simulink model "Progetto_robotics_linear"  (R2021a)
settings: Solver=ode4  StartTime=0.0  StopTime=Tsim_lin  FixedStep=Ts  RelTol=1e-3
InitFcn:
  | I1=1;
  | I2=2;
  | I3 =3;
values from neighbouring files (symbols this model uses):
  q_iniz_lin = [-pi/4;+3/4*pi;-3/4*pi]    [File_main_lineare.m]
(part 1 of 2)
settings Model: Creator=lorenzomaiani  LastModifiedBy=lorenzomaiani

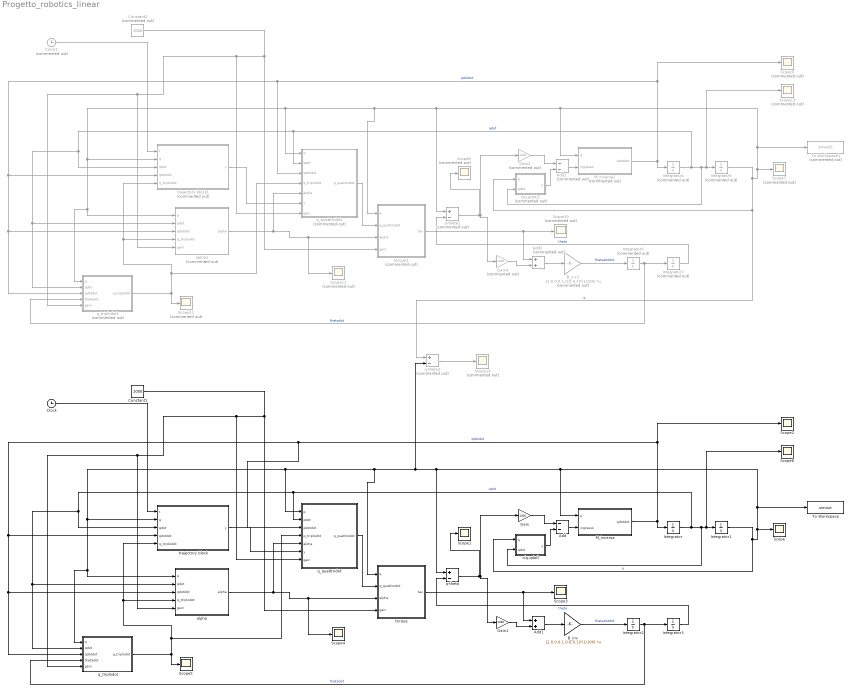
== system Progetto_robotics_linear ==
  "  M_inversa" : MATLAB Function  TreatAsAtomicUnit=on
  "  M_inversa1" : MATLAB Function  Commented=on  TreatAsAtomicUnit=on
  " c(q,qdot)" : MATLAB Function  TreatAsAtomicUnit=on
  " c(q,qdot)1" : MATLAB Function  Commented=on  TreatAsAtomicUnit=on
  Add : Sum  Inputs=--
  Add1 : Sum
  Add2 : Sum  Commented=on  Inputs=--
  Add3 : Sum  Commented=on
  B_inv : Gain  Gain=[1,0,0;0,1,0;0,0,1]*(1/100)  Multiplication=Matrix(K*u) (u vector)
  B_inv1 : Gain  Commented=on  Gain=[1,0,0;0,1,0;0,0,1]*(1/100)  Multiplication=Matrix(K*u) (u vector)
  Clock : Clock
  Clock1 : Clock  Commented=on
  Constant1 : Constant  Value=1000
  Constant2 : Constant  Commented=on  Value=1000
  Gain : Gain  Gain=1000
  Gain1 : Gain  Gain=1000
  Gain2 : Gain  Commented=on  Gain=1000
  Gain3 : Gain  Commented=on  Gain=1000
  Integrator : Integrator  InitialCondition=[0;0;0]
  Integrator1 : Integrator  InitialCondition=q_iniz_lin
  Integrator2 : Integrator  InitialCondition=[0;0;0]
  Integrator3 : Integrator  InitialCondition=q_iniz_lin
  Integrator4 : Integrator  Commented=on  InitialCondition=[0;0;0]
  Integrator5 : Integrator  Commented=on  InitialCondition=q_iniz_lin
  Integrator6 : Integrator  Commented=on  InitialCondition=[0;0;0]
  Integrator7 : Integrator  Commented=on  InitialCondition=q_iniz_lin
  Scope{,1..6} (7 alike) : Scope
  Scope{7..14} (8 alike) : Scope  Commented=on
  To Workspace : ToWorkspace  VariableName=simout  SampleTime=-1
  To Workspace1 : ToWorkspace  Commented=on  VariableName=simout1  SampleTime=-1
  alpha : MATLAB Function  TreatAsAtomicUnit=on
  alpha1 : MATLAB Function  Commented=on  TreatAsAtomicUnit=on
  q-theta : Sum  Inputs=+-
  q-theta1 : Sum  Commented=on  Inputs=+-
  q-theta2 : Sum  Commented=on  Inputs=+-
  q_quattrodot : MATLAB Function  TreatAsAtomicUnit=on
  q_quattrodot1 : MATLAB Function  Commented=on  TreatAsAtomicUnit=on
  q_triplodot : MATLAB Function  TreatAsAtomicUnit=on
  q_triplodot1 : MATLAB Function  Commented=on  TreatAsAtomicUnit=on
  torque : MATLAB Function  TreatAsAtomicUnit=on
  torque1 : MATLAB Function  Commented=on  TreatAsAtomicUnit=on
  trajectory block : MATLAB Function  TreatAsAtomicUnit=on
  trajectory block1 : MATLAB Function  Commented=on  TreatAsAtomicUnit=on
  wires:
  Integrator/1 -> q_quattrodot/2(qdot), q_triplodot/2(qdot), alpha/2(qdot), trajectory block/3(qdot), " c(q,qdot)"/2(qdot), Scope6/1, Integrator1/1  "qdot"
  Integrator1/1 -> To Workspace/1, "  M_inversa"/1(q), q-theta2/2, torque/1(q), q_quattrodot/1(q), alpha/1(q), q_triplodot/1(q), trajectory block/2(q), q-theta/1, Scope/1, " c(q,qdot)"/1(q)  "q"
  "  M_inversa"/1(qdotdot) -> Scope2/1, q_quattrodot/3(qdotdot), q_triplodot/3(qdotdot), alpha/3(qdotdot), trajectory block/4(qdotdot), Integrator/1  "qdotdot"
  " c(q,qdot)"/1(y) -> Add/2
  Gain/1 -> Add/1
  Integrator3/1 -> q-theta/2  "theta"
  Integrator2/1 -> q_triplodot/4(thetadot), Integrator3/1  "thetadot"
  Add1/1 -> B_inv/1
  Gain1/1 -> Add1/2
  q_quattrodot/1(q_quattrodot) -> torque/2(q_quattrodot)
  alpha/1(alpha) -> Scope4/1, torque/3(alpha), q_quattrodot/5(alpha)
  q_triplodot/1(q_triplodot) -> q_quattrodot/4(q_triplodot), trajectory block/5(q_triplodot), alpha/4(q_triplodot), Scope5/1
  trajectory block/1(y) -> q_quattrodot/6(y)
  Clock/1 -> trajectory block/1(t)
  Add/1 -> "  M_inversa"/2(ingresso)
  B_inv/1 -> Integrator2/1  "thetadotdot"
  Constant1/1 -> alpha/5(gain), q_triplodot/5(gain), q_quattrodot/7(gain), torque/4(gain)
  q-theta/1 -> Scope1/1, Gain/1, Gain1/1
  torque/1(tau) -> Scope3/1, Add1/1
  Gain2/1 -> Add2/1
  "  M_inversa1"/1(qdotdot) -> Scope9/1, q_quattrodot1/3(qdotdot), q_triplodot1/3(qdotdot), alpha1/3(qdotdot), trajectory block1/4(qdotdot), Integrator4/1  "qdotdot"
  alpha1/1(alpha) -> Scope11/1, torque1/3(alpha), q_quattrodot1/5(alpha)
  q-theta1/1 -> Scope8/1, Gain2/1, Gain3/1
  " c(q,qdot)1"/1(y) -> Add2/2
  Integrator7/1 -> q-theta1/2  "theta"
  Add3/1 -> B_inv1/1
  Constant2/1 -> alpha1/5(gain), q_triplodot1/5(gain), q_quattrodot1/7(gain), torque1/4(gain)
  Integrator5/1 -> To Workspace1/1, "  M_inversa1"/1(q), torque1/1(q), q_quattrodot1/1(q), alpha1/1(q), q_triplodot1/1(q), trajectory block1/2(q), q-theta1/1, Scope7/1, q-theta2/1, " c(q,qdot)1"/1(q)  "q"
  trajectory block1/1(y) -> q_quattrodot1/6(y)
  torque1/1(tau) -> Scope10/1, Add3/1
  Integrator6/1 -> q_triplodot1/4(thetadot), Integrator7/1  "thetadot"
  B_inv1/1 -> Integrator6/1  "thetadotdot"
  Integrator4/1 -> q_quattrodot1/2(qdot), q_triplodot1/2(qdot), alpha1/2(qdot), trajectory block1/3(qdot), " c(q,qdot)1"/2(qdot), Scope13/1, Integrator5/1  "qdot"
  q_triplodot1/1(q_triplodot) -> q_quattrodot1/4(q_triplodot), trajectory block1/5(q_triplodot), alpha1/4(q_triplodot), Scope12/1
  Gain3/1 -> Add3/2
  Clock1/1 -> trajectory block1/1(t)
  Add2/1 -> "  M_inversa1"/2(ingresso)
  q_quattrodot1/1(q_quattrodot) -> torque1/2(q_quattrodot)
  q-theta2/1 -> Scope14/1

== matlab function Progetto_robotics_linear/ c(q,qdot)1 ==
  data: q input; y output; qdot input
function y = fcn(q,qdot)


q1=q(1);
q2=q(2);
q3=q(3);

q1_dot=qdot(1);
q2_dot=qdot(2);
q3_dot=qdot(3);




c=[- q1_dot*(q3_dot*(5*sin(q2 + q3) + 5*sin(q3)) + q2_dot*(5*sin(q2 + q3) + 16*sin(q2))) - q3_dot*(q1_dot*(5*sin(q2 + q3) + 5*sin(q3)) + q2_dot*(5*sin(q2 + q3) + 5*sin(q3)) + q3_dot*(5*sin(q2 + q3) + 5*sin(q3))) - q2_dot*(q3_dot*(5*sin(q2 + q3) + 5*sin(q3)) + q2_dot*(5*sin(q2 + q3) + 11*sin(q2)) + q1_dot*(5*sin(q2 + q3) + 16*sin(q2)));
                                                                                                                                                                                q1_dot*(q1_dot*(5*sin(q2 + q3) + 16*sin(q2)) - 5*q3_dot*sin(q3)) - q3_dot*(5*q1_dot*sin(q3) + 5*q2_dot*sin(q3) + 10*q3_dot*sin(q3)) - 5*q2_dot*q3_dot*sin(q3);
                                                                                                                                                                                                                               q1_dot*(q1_dot*(5*sin(q2 + q3) + 5*sin(q3)) + 5*q2_dot*sin(q3)) + q2_dot*(5*q1_dot*sin(q3) + 5*q2_dot*sin(q3))];
                                                                                                                                                                                                                                                                                                                                                         
                                                                                                                                                                                                                                                                                                                                                            
                                                                                                                                                                                                                                                                                                                                                            
y = c;

== matlab function Progetto_robotics_linear/alpha1 ==
  data: q input; alpha output; qdot input; qdotdot input; q_triplodot input; gain input
function alpha = fcn(q,qdot,qdotdot,q_triplodot,gain)

q1=q(1);
q2=q(2);
q3=q(3);

q1_dot=qdot(1);
q2_dot=qdot(2);
q3_dot=qdot(3);

q1_dotdot=qdotdot(1);
q2_dotdot=qdotdot(2);
q3_dotdot=qdotdot(3);

%usare per blocco jacobiano
q1_tridot=q_triplodot(1);
q2_tridot=q_triplodot(2);
q3_tridot=q_triplodot(3);


K=gain*eye(3);
B=100*[1,0,0;0,1,0;0,0,1];


%M matrix
m=[10*cos(q2 + q3) + 32*cos(q2) + 10*cos(q3) + 5049/100, 5*cos(q2 + q3) + 11*cos(q2) + 10*cos(q3) + 504/25, 5*cos(q2 + q3) + 5*cos(q3) + 583/100;
   5*cos(q2 + q3) + 11*cos(q2) + 10*cos(q3) + 504/25,                              10*cos(q3) + 1133/50,                 10*cos(q3) + 583/100;
                5*cos(q2 + q3) + 5*cos(q3) + 583/100,                              10*cos(q3) + 583/100,                              583/100];



%coriolis and centrif.
c=[- q1_dot*(q3_dot*(5*sin(q2 + q3) + 5*sin(q3)) + q2_dot*(5*sin(q2 + q3) + 16*sin(q2))) - q3_dot*(q1_dot*(5*sin(q2 + q3) + 5*sin(q3)) + q2_dot*(5*sin(q2 + q3) + 5*sin(q3)) + q3_dot*(5*sin(q2 + q3) + 5*sin(q3))) - q2_dot*(q3_dot*(5*sin(q2 + q3) + 5*sin(q3)) + q2_dot*(5*sin(q2 + q3) + 11*sin(q2)) + q1_dot*(5*sin(q2 + q3) + 16*sin(q2)));
                                                                                                                                                                                q1_dot*(q1_dot*(5*sin(q2 + q3) + 16*sin(q2)) - 5*q3_dot*sin(q3)) - q3_dot*(5*q1_dot*sin(q3) + 5*q2_dot*sin(q3) + 10*q3_dot*sin(q3)) - 5*q2_dot*q3_dot*sin(q3);
                                                                                                                                                                                                                               q1_dot*(q1_dot*(5*sin(q2 + q3) + 5*sin(q3)) + 5*q2_dot*sin(q3)) + q2_dot*(5*q1_dot*sin(q3) + 5*q2_dot*sin(q3))];



%coriolis and centrif. dotdot
cdotdot=[11*q2_dot^4*sin(q2) + 5*q3_dot^4*sin(q3) - 22*q2_dotdot^2*sin(q2) - 10*q3_dotdot^2*sin(q3) + 5*q2_dot^4*sin(q2 + q3) + 5*q3_dot^4*sin(q2 + q3) - 10*q2_dotdot^2*sin(q2 + q3) - 10*q3_dotdot^2*sin(q2 + q3) - 32*q1_dot*q2_tridot*sin(q2) - 32*q2_dot*q1_tridot*sin(q2) - 22*q2_dot*q2_tridot*sin(q2) - 10*q1_dot*q3_tridot*sin(q3) - 10*q3_dot*q1_tridot*sin(q3) - 10*q2_dot*q3_tridot*sin(q3) - 10*q3_dot*q2_tridot*sin(q3) - 10*q3_dot*q3_tridot*sin(q3) - 64*q1_dotdot*q2_dotdot*sin(q2) - 20*q1_dotdot*q3_dotdot*sin(q3) - 20*q2_dotdot*q3_dotdot*sin(q3) - 20*q2_dot^2*q1_dotdot*cos(q2 + q3) - 25*q2_dot^2*q2_dotdot*cos(q2 + q3) - 20*q3_dot^2*q1_dotdot*cos(q2 + q3) - 25*q2_dot^2*q3_dotdot*cos(q2 + q3) - 25*q3_dot^2*q2_dotdot*cos(q2 + q3) - 25*q3_dot^2*q3_dotdot*cos(q2 + q3) + 10*q1_dot*q2_dot^3*sin(q2 + q3) + 10*q1_dot*q3_dot^3*sin(q2 + q3) + 20*q2_dot*q3_dot^3*sin(q2 + q3) + 20*q2_dot^3*q3_dot*sin(q2 + q3) - 64*q2_dot^2*q1_dotdot*cos(q2) - 55*q2_dot^2*q2_dotdot*cos(q2) - 20*q3_dot^2*q1_dotdot*cos(q3) - 20*q3_dot^2*q2_dotdot*cos(q3) - 25*q3_dot^2*q3_dotdot*cos(q3) + 32*q1_dot*q2_dot^3*sin(q2) + 10*q1_dot*q3_dot^3*sin(q3) + 10*q2_dot*q3_dot^3*sin(q3) + 30*q2_dot^2*q3_dot^2*sin(q2 + q3) - 10*q1_dot*q2_tridot*sin(q2 + q3) - 10*q2_dot*q1_tridot*sin(q2 + q3) - 10*q1_dot*q3_tridot*sin(q2 + q3) - 10*q2_dot*q2_tridot*sin(q2 + q3) - 10*q3_dot*q1_tridot*sin(q2 + q3) - 10*q2_dot*q3_tridot*sin(q2 + q3) - 10*q3_dot*q2_tridot*sin(q2 + q3) - 10*q3_dot*q3_tridot*sin(q2 + q3) - 20*q1_dotdot*q2_dotdot*sin(q2 + q3) - 20*q1_dotdot*q3_dotdot*sin(q2 + q3) - 20*q2_dotdot*q3_dotdot*sin(q2 + q3) - 30*q1_dot*q2_dot*q2_dotdot*cos(q2 + q3) - 30*q1_dot*q2_dot*q3_dotdot*cos(q2 + q3) - 30*q1_dot*q3_dot*q2_dotdot*cos(q2 + q3) - 40*q2_dot*q3_dot*q1_dotdot*cos(q2 + q3) - 30*q1_dot*q3_dot*q3_dotdot*cos(q2 + q3) - 50*q2_dot*q3_dot*q2_dotdot*cos(q2 + q3) - 50*q2_dot*q3_dot*q3_dotdot*cos(q2 + q3) - 96*q1_dot*q2_dot*q2_dotdot*cos(q2) - 30*q1_dot*q3_dot*q3_dotdot*cos(q3) - 30*q2_dot*q3_dot*q3_dotdot*cos(q3) + 30*q1_dot*q2_dot*q3_dot^2*sin(q2 + q3) + 30*q1_dot*q2_dot^2*q3_dot*sin(q2 + q3);
                                                                                                                                                                                                                                                                                                                                                                                                                                                                                                                                                                                                                                                                                                                                                                                                                                                                                                                                                                                                                                                                                                                                10*q3_dot^4*sin(q3) + 32*q1_dotdot^2*sin(q2) - 20*q3_dotdot^2*sin(q3) + 10*q1_dotdot^2*sin(q2 + q3) + 32*q1_dot*q1_tridot*sin(q2) - 10*q1_dot*q3_tridot*sin(q3) - 10*q3_dot*q1_tridot*sin(q3) - 10*q2_dot*q3_tridot*sin(q3) - 10*q3_dot*q2_tridot*sin(q3) - 20*q3_dot*q3_tridot*sin(q3) - 20*q1_dotdot*q3_dotdot*sin(q3) - 20*q2_dotdot*q3_dotdot*sin(q3) + 5*q1_dot^2*q2_dotdot*cos(q2 + q3) + 5*q1_dot^2*q3_dotdot*cos(q2 + q3) + 16*q1_dot^2*q2_dotdot*cos(q2) - 20*q3_dot^2*q1_dotdot*cos(q3) - 20*q3_dot^2*q2_dotdot*cos(q3) - 50*q3_dot^2*q3_dotdot*cos(q3) + 10*q1_dot*q3_dot^3*sin(q3) + 10*q2_dot*q3_dot^3*sin(q3) - 5*q1_dot^2*q2_dot^2*sin(q2 + q3) - 5*q1_dot^2*q3_dot^2*sin(q2 + q3) - 16*q1_dot^2*q2_dot^2*sin(q2) + 10*q1_dot*q1_tridot*sin(q2 + q3) + 20*q1_dot*q2_dot*q1_dotdot*cos(q2 + q3) + 20*q1_dot*q3_dot*q1_dotdot*cos(q2 + q3) + 64*q1_dot*q2_dot*q1_dotdot*cos(q2) - 30*q1_dot*q3_dot*q3_dotdot*cos(q3) - 30*q2_dot*q3_dot*q3_dotdot*cos(q3) - 10*q1_dot^2*q2_dot*q3_dot*sin(q2 + q3);
                                                                                                                                                                                                                                                                                                                                                                                                                                                                                                                                                                                                                                                                                                                                                                                                                                                                                                                                                                                                                                                                                                                                                                                                                                                                                                                                                                                        10*q2_dotdot^2*sin(q3) + q1_tridot*(10*q1_dot*sin(q2 + q3) + 10*q1_dot*sin(q3) + 10*q2_dot*sin(q3)) + q3_dotdot*(5*q1_dot^2*cos(q3) + 5*q2_dot^2*cos(q3) + 5*q1_dot^2*cos(q2 + q3) + 10*q1_dot*q2_dot*cos(q3)) - q3_dot^2*(5*q1_dot^2*sin(q3) + 5*q2_dot^2*sin(q3) + 5*q1_dot^2*sin(q2 + q3) + 10*q1_dot*q2_dot*sin(q3)) + q1_dotdot^2*(10*sin(q2 + q3) + 10*sin(q3)) + 20*q1_dotdot*q2_dotdot*sin(q3) + 5*q1_dot^2*q2_dotdot*cos(q2 + q3) + 2*q3_dot*q1_dotdot*(10*q1_dot*cos(q2 + q3) + 10*q1_dot*cos(q3) + 10*q2_dot*cos(q3)) + q2_tridot*sin(q3)*(10*q1_dot + 10*q2_dot) - 5*q1_dot^2*q2_dot^2*sin(q2 + q3) + 2*q3_dot*q2_dotdot*cos(q3)*(10*q1_dot + 10*q2_dot) + 20*q1_dot*q2_dot*q1_dotdot*cos(q2 + q3) - 10*q1_dot^2*q2_dot*q3_dot*sin(q2 + q3)];
                                                                                                                                                                                                                                                                                                                                                                                                          
 




mdot=[- q3_dot*(10*sin(q2 + q3) + 10*sin(q3)) - q2_dot*(10*sin(q2 + q3) + 32*sin(q2)), - q2_dot*(5*sin(q2 + q3) + 11*sin(q2)) - q3_dot*(5*sin(q2 + q3) + 10*sin(q3)), - 5*q2_dot*sin(q2 + q3) - q3_dot*(5*sin(q2 + q3) + 5*sin(q3));
  - q2_dot*(5*sin(q2 + q3) + 11*sin(q2)) - q3_dot*(5*sin(q2 + q3) + 10*sin(q3)),                                                            -10*q3_dot*sin(q3),                                            -10*q3_dot*sin(q3);
                 - 5*q2_dot*sin(q2 + q3) - q3_dot*(5*sin(q2 + q3) + 5*sin(q3)),                                                            -10*q3_dot*sin(q3),                                                             0];
 

mdotdot=[(- 10*cos(q2 + q3) - 32*cos(q2))*q2_dot^2 - 20*cos(q2 + q3)*q2_dot*q3_dot + (- 10*cos(q2 + q3) - 10*cos(q3))*q3_dot^2 - q3_dotdot*(10*sin(q2 + q3) + 10*sin(q3)) - q2_dotdot*(10*sin(q2 + q3) + 32*sin(q2)), (- 5*cos(q2 + q3) - 11*cos(q2))*q2_dot^2 - 10*cos(q2 + q3)*q2_dot*q3_dot + (- 5*cos(q2 + q3) - 10*cos(q3))*q3_dot^2 - q2_dotdot*(5*sin(q2 + q3) + 11*sin(q2)) - q3_dotdot*(5*sin(q2 + q3) + 10*sin(q3)), - 5*cos(q2 + q3)*q2_dot^2 - 10*cos(q2 + q3)*q2_dot*q3_dot + (- 5*cos(q2 + q3) - 5*cos(q3))*q3_dot^2 - 5*q2_dotdot*sin(q2 + q3) - q3_dotdot*(5*sin(q2 + q3) + 5*sin(q3));
    (- 5*cos(q2 + q3) - 11*cos(q2))*q2_dot^2 - 10*cos(q2 + q3)*q2_dot*q3_dot + (- 5*cos(q2 + q3) - 10*cos(q3))*q3_dot^2 - q2_dotdot*(5*sin(q2 + q3) + 11*sin(q2)) - q3_dotdot*(5*sin(q2 + q3) + 10*sin(q3)),                                                                                                                                                            - 10*cos(q3)*q3_dot^2 - 10*q3_dotdot*sin(q3),                                                                                                                            - 10*cos(q3)*q3_dot^2 - 10*q3_dotdot*sin(q3);
                                    - 5*cos(q2 + q3)*q2_dot^2 - 10*cos(q2 + q3)*q2_dot*q3_dot + (- 5*cos(q2 + q3) - 5*cos(q3))*q3_dot^2 - 5*q2_dotdot*sin(q2 + q3) - q3_dotdot*(5*sin(q2 + q3) + 5*sin(q3)),                                                                                                                                                            - 10*cos(q3)*q3_dot^2 - 10*q3_dotdot*sin(q3),                                                                                                                                                                       0];
 
                                    
alpha = 2*mdot*[q1_tridot;q2_tridot;q3_tridot]+(mdotdot+K+K*inv(B)*m)*[q1_dotdot;q2_dotdot;q3_dotdot]+cdotdot+c ;

== matlab function Progetto_robotics_linear/q_quattrodot1 ==
  data: q input; qdot input; qdotdot input; q_triplodot input; alpha input; q_quattrodot output; y input; gain input
% THIS CODE COMPUTES THE FOURTH DERIVATIVE OF THE JOINT VARIABLES q BASED
% ON A CONSTRAINED OPTIMIZATION ALGORITHM

% UNCOMMENT EACH SECTION CORRESPONDING TO THE FOLLOWING SUBDIVISIONS

% CASE A1:   W=I   , tau_0=0
% CASE B1:   W=inv(M)   , tau_0=0
% CASE C1:   W=inv(M)^2   , tau_0=0

% CASE A2:   W=I   , tau_0!=0
% CASE B2:   W=inv(M)   , tau_0!=0
% CASE C2:   W=inv(M)^2   , tau_0!=0

%% CASE A1

% function q_quattrodot = fcn(q,qdot,qdotdot,q_triplodot,alpha,y,gain)
% 
% q1=q(1);
% q2=q(2);
% q3=q(3);
% 
% q1_dot=qdot(1);
% q2_dot=qdot(2);
% q3_dot=qdot(3);
% 
% q1_dotdot=qdotdot(1);
% q2_dotdot=qdotdot(2);
% q3_dotdot=qdotdot(3);
% 
% q1_tridot=q_triplodot(1);
% q2_tridot=q_triplodot(2);
% q3_tridot=q_triplodot(3);
% 
% K=gain*[1,0,0;
%     0,1,0;
%     0,0,1];
% B=100*[1,0,0;
%     0,1,0;
%     0,0,1];
% 
% 
% M=[10*cos(q2 + q3) + 32*cos(q2) + 10*cos(q3) + 5049/100, 5*cos(q2 + q3) + 11*cos(q2) + 10*cos(q3) + 504/25, 5*cos(q2 + q3) + 5*cos(q3) + 583/100;
%    5*cos(q2 + q3) + 11*cos(q2) + 10*cos(q3) + 504/25,                              10*cos(q3) + 1133/50,                 10*cos(q3) + 583/100;
%                 5*cos(q2 + q3) + 5*cos(q3) + 583/100,                              10*cos(q3) + 583/100,                              583/100];
%               
%              
% 
%              
% J=[- sin(q1 + q2 + q3) - sin(q1 + q2) - sin(q1), - sin(q1 + q2 + q3) - sin(q1 + q2), -sin(q1 + q2 + q3);
%  cos(q1 + q2 + q3) + cos(q1 + q2) + cos(q1),   cos(q1 + q2 + q3) + cos(q1 + q2),  cos(q1 + q2 + q3)];
% 
% A=B*inv(K);
% W1=M*A^2*M;
% Jpinv=inv(W1)*transpose(J)*inv(J*inv(W1)*transpose(J)); 
% 
% q_quattrodot =-(eye(3)-Jpinv*J)*inv(M)*alpha + Jpinv *y;
% 


%% CASE B1
% 
% function q_quattrodot = fcn(q,qdot,qdotdot,q_triplodot,alpha,y,gain)
% 
% q1=q(1);
% q2=q(2);
% q3=q(3);
% 
% % q1_dot=qdot(1);
% % q2_dot=qdot(2);
% % q3_dot=qdot(3);
% % 
% % q1_dotdot=qdotdot(1);
% % q2_dotdot=qdotdot(2);
% % q3_dotdot=qdotdot(3);
% % 
% % q1_tridot=q_triplodot(1);
% % q2_tridot=q_triplodot(2);
% % q3_tridot=q_triplodot(3);
% 
% K=gain*[1,0,0;
%     0,1,0;
%     0,0,1];
% B=100*[1,0,0;
%     0,1,0;
%     0,0,1];
% 
% 
% M=[10*cos(q2 + q3) + 32*cos(q2) + 10*cos(q3) + 5049/100, 5*cos(q2 + q3) + 11*cos(q2) + 10*cos(q3) + 504/25, 5*cos(q2 + q3) + 5*cos(q3) + 583/100;
%    5*cos(q2 + q3) + 11*cos(q2) + 10*cos(q3) + 504/25,                              10*cos(q3) + 1133/50,                 10*cos(q3) + 583/100;
%                 5*cos(q2 + q3) + 5*cos(q3) + 583/100,                              10*cos(q3) + 583/100,                              583/100];
%               
%              
% 
%              
% J=[- sin(q1 + q2 + q3) - sin(q1 + q2) - sin(q1), - sin(q1 + q2 + q3) - sin(q1 + q2), -sin(q1 + q2 + q3);
%  cos(q1 + q2 + q3) + cos(q1 + q2) + cos(q1),   cos(q1 + q2 + q3) + cos(q1 + q2),  cos(q1 + q2 + q3)];
% 
% % questa è la soluzione di donato
% q_quattrodot =-inv(M)*alpha+inv(M)*transpose(J)*inv(J*transpose(J))*J*alpha+transpose(J)*inv(J*transpose(J))*y;






%% CASE C1
% function q_quattrodot = fcn(q,qdot,qdotdot,q_triplodot,alpha,y,gain)
% 
% q1=q(1);
% q2=q(2);
% q3=q(3);
% 
% q1_dot=qdot(1);
% q2_dot=qdot(2);
% q3_dot=qdot(3);
% 
% q1_dotdot=qdotdot(1);
% q2_dotdot=qdotdot(2);
% q3_dotdot=qdotdot(3);
% 
% q1_tridot=q_triplodot(1);
% q2_tridot=q_triplodot(2);
% q3_tridot=q_triplodot(3);
% 
% K=gain*[1,0,0;
%     0,1,0;
%     0,0,1];
% B=100*[1,0,0;
%     0,1,0;
%     0,0,1];
% 
% 
% M=[10*cos(q2 + q3) + 32*cos(q2) + 10*cos(q3) + 5049/100, 5*cos(q2 + q3) + 11*cos(q2) + 10*cos(q3) + 504/25, 5*cos(q2 + q3) + 5*cos(q3) + 583/100;
%    5*cos(q2 + q3) + 11*cos(q2) + 10*cos(q3) + 504/25,                              10*cos(q3) + 1133/50,                 10*cos(q3) + 583/100;
%                 5*cos(q2 + q3) + 5*cos(q3) + 583/100,                              10*cos(q3) + 583/100,                              583/100];
%               
%              
% 
%              
% J=[- sin(q1 + q2 + q3) - sin(q1 + q2) - sin(q1), - sin(q1 + q2 + q3) - sin(q1 + q2), -sin(q1 + q2 + q3);
%  cos(q1 + q2 + q3) + cos(q1 + q2) + cos(q1),   cos(q1 + q2 + q3) + cos(q1 + q2),  cos(q1 + q2 + q3)];
% 
% 
% q_quattrodot =-inv(M)*alpha+inv(M)*transpose(J)*inv(J*transpose(J))*J*alpha+transpose(J)*inv(J*transpose(J))*y;

          
%% CASE A2
% function q_quattrodot = fcn(q,qdot,qdotdot,q_triplodot,alpha,y,gain)
% 
% q1=q(1);
% q2=q(2);
% q3=q(3);
% 
% q1_dot=qdot(1);
% q2_dot=qdot(2);
% q3_dot=qdot(3);
% 
% q1_dotdot=qdotdot(1);
% q2_dotdot=qdotdot(2);
% q3_dotdot=qdotdot(3);
% 
% q1_tridot=q_triplodot(1);
% q2_tridot=q_triplodot(2);
% q3_tridot=q_triplodot(3);
% 
% K=gain*[1,0,0;
%     0,1,0;
%     0,0,1];
% B=100*[1,0,0;
%     0,1,0;
%     0,0,1];
% 
% 
% M=[10*cos(q2 + q3) + 32*cos(q2) + 10*cos(q3) + 5049/100, 5*cos(q2 + q3) + 16*cos(q2) + 10*cos(q3) + 1133/50, 5*cos(q2 + q3) + 5*cos(q3) + 583/100;
%   5*cos(q2 + q3) + 16*cos(q2) + 10*cos(q3) + 1133/50,                               10*cos(q3) + 1133/50,                  5*cos(q3) + 583/100;
%                5*cos(q2 + q3) + 5*cos(q3) + 583/100,                                5*cos(q3) + 583/100,                              583/100];
% 
% J=[- sin(q1 + q2 + q3) - sin(q1 + q2) - sin(q1), - sin(q1 + q2 + q3) - sin(q1 + q2), -sin(q1 + q2 + q3);
%  cos(q1 + q2 + q3) + cos(q1 + q2) + cos(q1),   cos(q1 + q2 + q3) + cos(q1 + q2),  cos(q1 + q2 + q3)];
%               
%              
% 
% K_1=125*eye(3);             
% K_2=75*eye(3);      
% K_3=25*eye(3);    
% 
% tau_0=-K_1*[q1_dot;q2_dot;q3_dot]-K_2*[q1_dotdot;q2_dotdot;q3_dotdot]-K_3*[q1_tridot;q2_tridot;q3_tridot];       
% 
% A=B*inv(K);
%              
% Jpinv=inv(M*A^2*M)*transpose(J)*inv(J*inv(M*A^2*M)*transpose(J));
% 
% q_quattrodot =(eye(3)-Jpinv *J)*inv(M)*inv(A)*tau_0-(eye(3)-Jpinv *J)*inv(M)*alpha+Jpinv*y;       
% 
% 
% 
%% CASE B2
% 
function q_quattrodot = fcn(q,qdot,qdotdot,q_triplodot,alpha,y,gain)

q1=q(1);
q2=q(2);
q3=q(3);

q1_dot=qdot(1);
q2_dot=qdot(2);
q3_dot=qdot(3);

q1_dotdot=qdotdot(1);
q2_dotdot=qdotdot(2);
q3_dotdot=qdotdot(3);

q1_tridot=q_triplodot(1);
q2_tridot=q_triplodot(2);
q3_tridot=q_triplodot(3);

K=gain*[1,0,0;
    0,1,0;
    0,0,1];
B=100*[1,0,0;
    0,1,0;
    0,0,1];


M=[10*cos(q2 + q3) + 32*cos(q2) + 10*cos(q3) + 5049/100, 5*cos(q2 + q3) + 16*cos(q2) + 10*cos(q3) + 1133/50, 5*cos(q2 + q3) + 5*cos(q3) + 583/100;
  5*cos(q2 + q3) + 16*cos(q2) + 10*cos(q3) + 1133/50,                               10*cos(q3) + 1133/50,                  5*cos(q3) + 583/100;
               5*cos(q2 + q3) + 5*cos(q3) + 583/100,                                5*cos(q3) + 583/100,                              583/100];

J=[- sin(q1 + q2 + q3) - sin(q1 + q2) - sin(q1), - sin(q1 + q2 + q3) - sin(q1 + q2), -sin(q1 + q2 + q3);
 cos(q1 + q2 + q3) + cos(q1 + q2) + cos(q1),   cos(q1 + q2 + q3) + cos(q1 + q2),  cos(q1 + q2 + q3)];


% K_1=125*eye(3);             
% K_2=75*eye(3);      
% K_3=25*eye(3); 

% (s+10)^3
K_1=1000*eye(3);             
K_2=300*eye(3);      
K_3=30*eye(3);

tau_0=-K_1*[q1_dot;q2_dot;q3_dot]-K_2*[q1_dotdot;q2_dotdot;q3_dotdot]-K_3*[q1_tridot;q2_tridot;q3_tridot];       

% soluzione donato
%q_quattrodot=-inv(M)*alpha+inv(M*B*inv(K))*tau_0+inv(M)*transpose(J)*inv(J*transpose(J))*J*alpha-inv(M*B*inv(K))*transpose(J)*inv(J*transpose(J))*J*tau_0+transpose(J)*inv(J*transpose(J))*y;

J_pinv_minv=inv(M)*transpose(J)*inv(J*inv(M)*transpose(J));
q_quattrodot =(J_pinv_minv*J-eye(3))*inv(M)*alpha+J_pinv_minv*y+(eye(3)-J_pinv_minv*J)*inv(M)*inv(B*inv(K))*tau_0;


% 
%% CASE C2
% 
% function q_quattrodot = fcn(q,qdot,qdotdot,q_triplodot,alpha,y,gain)
% 
% q1=q(1);
% q2=q(2);
% q3=q(3);
% 
% q1_dot=qdot(1);
% q2_dot=qdot(2);
% q3_dot=qdot(3);
% 
% q1_dotdot=qdotdot(1);
% q2_dotdot=qdotdot(2);
% q3_dotdot=qdotdot(3);
% 
% q1_tridot=q_triplodot(1);
% q2_tridot=q_triplodot(2);
% q3_tridot=q_triplodot(3);
% 
% K=gain*[1,0,0;
%     0,1,0;
%     0,0,1];
% B=100*[1,0,0;
%     0,1,0;
%     0,0,1];
% 
% 
% M=[10*cos(q2 + q3) + 32*cos(q2) + 10*cos(q3) + 5049/100, 5*cos(q2 + q3) + 16*cos(q2) + 10*cos(q3) + 1133/50, 5*cos(q2 + q3) + 5*cos(q3) + 583/100;
%   5*cos(q2 + q3) + 16*cos(q2) + 10*cos(q3) + 1133/50,                               10*cos(q3) + 1133/50,                  5*cos(q3) + 583/100;
%                5*cos(q2 + q3) + 5*cos(q3) + 583/100,                                5*cos(q3) + 583/100,                              583/100];
% 
% J=[- sin(q1 + q2 + q3) - sin(q1 + q2) - sin(q1), - sin(q1 + q2 + q3) - sin(q1 + q2), -sin(q1 + q2 + q3);
%  cos(q1 + q2 + q3) + cos(q1 + q2) + cos(q1),   cos(q1 + q2 + q3) + cos(q1 + q2),  cos(q1 + q2 + q3)];
%               
% 
% K_1=125*eye(3);             
% K_2=75*eye(3);      
% K_3=25*eye(3);    
% 
%  tau_0=-K_1*[q1_dot;q2_dot;q3_dot]-K_2*[q1_dotdot;q2_dotdot;q3_dotdot]-K_3*[q1_tridot;q2_tridot;q3_tridot];       
% 
% q_quattrodot=-inv(M)*alpha+inv(B*inv(K)*M)*tau_0-transpose(J)*inv(J*transpose(J))*(-J*inv(M)*alpha+J*inv(B*inv(K)*M)*tau_0-y);

== matlab function Progetto_robotics_linear/q_triplodot1 ==
  data: q input; q_triplodot output; qdot input; qdotdot input; thetadot input; gain input
function q_triplodot = fcn(q,qdot,qdotdot,thetadot,gain)




q1=q(1);
q2=q(2);
q3=q(3);

q1_dot=qdot(1);
q2_dot=qdot(2);
q3_dot=qdot(3);

q1_dotdot=qdotdot(1);
q2_dotdot=qdotdot(2);
q3_dotdot=qdotdot(3);

tdot=[thetadot(1);thetadot(2);thetadot(3)];





%elastic matrix
K=gain*eye(3);


%M matrix
m=[10*cos(q2 + q3) + 32*cos(q2) + 10*cos(q3) + 5049/100, 5*cos(q2 + q3) + 11*cos(q2) + 10*cos(q3) + 504/25, 5*cos(q2 + q3) + 5*cos(q3) + 583/100;
   5*cos(q2 + q3) + 11*cos(q2) + 10*cos(q3) + 504/25,                              10*cos(q3) + 1133/50,                 10*cos(q3) + 583/100;
                5*cos(q2 + q3) + 5*cos(q3) + 583/100,                              10*cos(q3) + 583/100,                              583/100];


%coriolis and centrif. dot
cdot=[- 11*q2_dot^3*cos(q2) - 5*q3_dot^3*cos(q3) - 5*q2_dot^3*cos(q2 + q3) - 5*q3_dot^3*cos(q2 + q3) - 32*q1_dot*q2_dotdot*sin(q2) - 32*q2_dot*q1_dotdot*sin(q2) - 22*q2_dot*q2_dotdot*sin(q2) - 10*q1_dot*q3_dotdot*sin(q3) - 10*q3_dot*q1_dotdot*sin(q3) - 10*q2_dot*q3_dotdot*sin(q3) - 10*q3_dot*q2_dotdot*sin(q3) - 10*q3_dot*q3_dotdot*sin(q3) - 10*q1_dot*q2_dot^2*cos(q2 + q3) - 10*q1_dot*q3_dot^2*cos(q2 + q3) - 15*q2_dot*q3_dot^2*cos(q2 + q3) - 15*q2_dot^2*q3_dot*cos(q2 + q3) - 32*q1_dot*q2_dot^2*cos(q2) - 10*q1_dot*q3_dot^2*cos(q3) - 10*q2_dot*q3_dot^2*cos(q3) - 10*q1_dot*q2_dotdot*sin(q2 + q3) - 10*q2_dot*q1_dotdot*sin(q2 + q3) - 10*q1_dot*q3_dotdot*sin(q2 + q3) - 10*q2_dot*q2_dotdot*sin(q2 + q3) - 10*q3_dot*q1_dotdot*sin(q2 + q3) - 10*q2_dot*q3_dotdot*sin(q2 + q3) - 10*q3_dot*q2_dotdot*sin(q2 + q3) - 10*q3_dot*q3_dotdot*sin(q2 + q3) - 20*q1_dot*q2_dot*q3_dot*cos(q2 + q3);
                                                                                                                                                                                                                                                                                                                                                                                                                                                                                                         32*q1_dot*q1_dotdot*sin(q2) - 10*q3_dot^3*cos(q3) - 10*q1_dot*q3_dotdot*sin(q3) - 10*q3_dot*q1_dotdot*sin(q3) - 10*q2_dot*q3_dotdot*sin(q3) - 10*q3_dot*q2_dotdot*sin(q3) - 20*q3_dot*q3_dotdot*sin(q3) + 5*q1_dot^2*q2_dot*cos(q2 + q3) + 5*q1_dot^2*q3_dot*cos(q2 + q3) + 16*q1_dot^2*q2_dot*cos(q2) - 10*q1_dot*q3_dot^2*cos(q3) - 10*q2_dot*q3_dot^2*cos(q3) + 10*q1_dot*q1_dotdot*sin(q2 + q3);
                                                                                                                                                                                                                                                                                                                                                                                                                                                                                                                                                                                                                        q1_dotdot*(2*q1_dot*(5*sin(q2 + q3) + 5*sin(q3)) + 10*q2_dot*sin(q3)) + q2_dotdot*(10*q1_dot*sin(q3) + 10*q2_dot*sin(q3)) + q3_dot*(q1_dot*(q1_dot*(5*cos(q2 + q3) + 5*cos(q3)) + 5*q2_dot*cos(q3)) + q2_dot*(5*q1_dot*cos(q3) + 5*q2_dot*cos(q3))) + 5*q1_dot^2*q2_dot*cos(q2 + q3)];
 
  
                                                                                                                                                                                                    

mdot=[- q3_dot*(10*sin(q2 + q3) + 10*sin(q3)) - q2_dot*(10*sin(q2 + q3) + 32*sin(q2)), - q2_dot*(5*sin(q2 + q3) + 11*sin(q2)) - q3_dot*(5*sin(q2 + q3) + 10*sin(q3)), - 5*q2_dot*sin(q2 + q3) - q3_dot*(5*sin(q2 + q3) + 5*sin(q3));
  - q2_dot*(5*sin(q2 + q3) + 11*sin(q2)) - q3_dot*(5*sin(q2 + q3) + 10*sin(q3)),                                                            -10*q3_dot*sin(q3),                                            -10*q3_dot*sin(q3);
                 - 5*q2_dot*sin(q2 + q3) - q3_dot*(5*sin(q2 + q3) + 5*sin(q3)),                                                            -10*q3_dot*sin(q3),                                                             0];


q_triplodot = -inv(m)*(mdot*[q1_dotdot;q2_dotdot;q3_dotdot]+cdot+K*([q1_dot;q2_dot;q3_dot]-tdot));

== matlab function Progetto_robotics_linear/torque1 ==
  data: q input; tau output; q_quattrodot input; alpha input; gain input
function tau = fcn(q,q_quattrodot,alpha,gain)
B=100*[1,0,0;
    0,1,0;
    0,0,1];
K=gain*eye(3);

q1=q(1);
q2=q(2);
q3=q(3);

M=[10*cos(q2 + q3) + 32*cos(q2) + 10*cos(q3) + 5049/100, 5*cos(q2 + q3) + 11*cos(q2) + 10*cos(q3) + 504/25, 5*cos(q2 + q3) + 5*cos(q3) + 583/100;
   5*cos(q2 + q3) + 11*cos(q2) + 10*cos(q3) + 504/25,                              10*cos(q3) + 1133/50,                 10*cos(q3) + 583/100;
                5*cos(q2 + q3) + 5*cos(q3) + 583/100,                              10*cos(q3) + 583/100,                              583/100];




tau = B*inv(K)*(M*q_quattrodot+alpha);

== matlab function Progetto_robotics_linear/trajectory block1 ==
  data: t input; y output; q input; qdot input; qdotdot input; q_triplodot input
function y = fcn(t,q,qdot,qdotdot,q_triplodot)



q1=q(1);
q2=q(2);
q3=q(3);

q1_dot=qdot(1);
q2_dot=qdot(2);
q3_dot=qdot(3);

q1_dotdot=qdotdot(1);
q2_dotdot=qdotdot(2);
q3_dotdot=qdotdot(3);


q1_tridot=q_triplodot(1);
q2_tridot=q_triplodot(2);
q3_tridot=q_triplodot(3);


p=[cos(q1)+cos(q1+q2)+cos(q1+q2+q3);
    sin(q1)+sin(q1+q2)+sin(q1+q2+q3)];


%JACOBIANO
J=[- sin(q1 + q2 + q3) - sin(q1 + q2) - sin(q1), - sin(q1 + q2 + q3) - sin(q1 + q2), -sin(q1 + q2 + q3);
 cos(q1 + q2 + q3) + cos(q1 + q2) + cos(q1),   cos(q1 + q2 + q3) + cos(q1 + q2),  cos(q1 + q2 + q3)];


%JDOT
Jdot=[- q1_dot*(cos(q1 + q2 + q3) + cos(q1 + q2) + cos(q1)) - q3_dot*cos(q1 + q2 + q3) - q2_dot*(cos(q1 + q2 + q3) + cos(q1 + q2)), - q3_dot*cos(q1 + q2 + q3) - q1_dot*(cos(q1 + q2 + q3) + cos(q1 + q2)) - q2_dot*(cos(q1 + q2 + q3) + cos(q1 + q2)), -cos(q1 + q2 + q3)*(q1_dot + q2_dot + q3_dot);
- q2_dot*(sin(q1 + q2 + q3) + sin(q1 + q2)) - q1_dot*(sin(q1 + q2 + q3) + sin(q1 + q2) + sin(q1)) - q3_dot*sin(q1 + q2 + q3), - q1_dot*(sin(q1 + q2 + q3) + sin(q1 + q2)) - q2_dot*(sin(q1 + q2 + q3) + sin(q1 + q2)) - q3_dot*sin(q1 + q2 + q3), -sin(q1 + q2 + q3)*(q1_dot + q2_dot + q3_dot)];
 

%JDOTDOT
Jdotdot=[  q1_dot^2*(sin(q1 + q2 + q3) + sin(q1 + q2) + sin(q1)) + q3_dot^2*sin(q1 + q2 + q3) + q2_dot^2*(sin(q1 + q2 + q3) + sin(q1 + q2)) - q1_dotdot*(cos(q1 + q2 + q3) + cos(q1 + q2) + cos(q1)) - q3_dotdot*cos(q1 + q2 + q3) - q2_dotdot*(cos(q1 + q2 + q3) + cos(q1 + q2)) + 2*q1_dot*q3_dot*sin(q1 + q2 + q3) + 2*q2_dot*q3_dot*sin(q1 + q2 + q3) + 2*q1_dot*q2_dot*(sin(q1 + q2 + q3) + sin(q1 + q2)),   q3_dot^2*sin(q1 + q2 + q3) + q1_dot^2*(sin(q1 + q2 + q3) + sin(q1 + q2)) + q2_dot^2*(sin(q1 + q2 + q3) + sin(q1 + q2)) - q3_dotdot*cos(q1 + q2 + q3) - q1_dotdot*(cos(q1 + q2 + q3) + cos(q1 + q2)) - q2_dotdot*(cos(q1 + q2 + q3) + cos(q1 + q2)) + 2*q1_dot*q3_dot*sin(q1 + q2 + q3) + 2*q2_dot*q3_dot*sin(q1 + q2 + q3) + 2*q1_dot*q2_dot*(sin(q1 + q2 + q3) + sin(q1 + q2)),   sin(q1 + q2 + q3)*q1_dot^2 + 2*sin(q1 + q2 + q3)*q1_dot*q2_dot + 2*sin(q1 + q2 + q3)*q1_dot*q3_dot + sin(q1 + q2 + q3)*q2_dot^2 + 2*sin(q1 + q2 + q3)*q2_dot*q3_dot + sin(q1 + q2 + q3)*q3_dot^2 - q1_dotdot*cos(q1 + q2 + q3) - q2_dotdot*cos(q1 + q2 + q3) - q3_dotdot*cos(q1 + q2 + q3);
- q2_dotdot*(sin(q1 + q2 + q3) + sin(q1 + q2)) - q1_dot^2*(cos(q1 + q2 + q3) + cos(q1 + q2) + cos(q1)) - q3_dot^2*cos(q1 + q2 + q3) - q2_dot^2*(cos(q1 + q2 + q3) + cos(q1 + q2)) - q1_dotdot*(sin(q1 + q2 + q3) + sin(q1 + q2) + sin(q1)) - q3_dotdot*sin(q1 + q2 + q3) - 2*q1_dot*q3_dot*cos(q1 + q2 + q3) - 2*q2_dot*q3_dot*cos(q1 + q2 + q3) - 2*q1_dot*q2_dot*(cos(q1 + q2 + q3) + cos(q1 + q2)), - q1_dotdot*(sin(q1 + q2 + q3) + sin(q1 + q2)) - q2_dotdot*(sin(q1 + q2 + q3) + sin(q1 + q2)) - q3_dot^2*cos(q1 + q2 + q3) - q1_dot^2*(cos(q1 + q2 + q3) + cos(q1 + q2)) - q2_dot^2*(cos(q1 + q2 + q3) + cos(q1 + q2)) - q3_dotdot*sin(q1 + q2 + q3) - 2*q1_dot*q3_dot*cos(q1 + q2 + q3) - 2*q2_dot*q3_dot*cos(q1 + q2 + q3) - 2*q1_dot*q2_dot*(cos(q1 + q2 + q3) + cos(q1 + q2)), - cos(q1 + q2 + q3)*q1_dot^2 - 2*cos(q1 + q2 + q3)*q1_dot*q2_dot - 2*cos(q1 + q2 + q3)*q1_dot*q3_dot - cos(q1 + q2 + q3)*q2_dot^2 - 2*cos(q1 + q2 + q3)*q2_dot*q3_dot - cos(q1 + q2 + q3)*q3_dot^2 - q1_dotdot*sin(q1 + q2 + q3) - q2_dotdot*sin(q1 + q2 + q3) - q3_dotdot*sin(q1 + q2 + q3)];
 
%JTRIPLODOT
Jtriplodot=[q1_dot^3*cos(q1) + q1_dot^3*cos(q1 + q2 + q3) + q2_dot^3*cos(q1 + q2 + q3) + q3_dot^3*cos(q1 + q2 + q3) - q1_tridot*cos(q1 + q2) - q2_tridot*cos(q1 + q2) - q1_tridot*cos(q1) + q1_dot^3*cos(q1 + q2) + q2_dot^3*cos(q1 + q2) - q1_tridot*cos(q1 + q2 + q3) - q2_tridot*cos(q1 + q2 + q3) - q3_tridot*cos(q1 + q2 + q3) + 3*q1_dot*q1_dotdot*sin(q1) + 3*q1_dot*q2_dot^2*cos(q1 + q2) + 3*q1_dot^2*q2_dot*cos(q1 + q2) + 3*q1_dot*q1_dotdot*sin(q1 + q2 + q3) + 3*q1_dot*q2_dotdot*sin(q1 + q2 + q3) + 3*q2_dot*q1_dotdot*sin(q1 + q2 + q3) + 3*q1_dot*q3_dotdot*sin(q1 + q2 + q3) + 3*q2_dot*q2_dotdot*sin(q1 + q2 + q3) + 3*q3_dot*q1_dotdot*sin(q1 + q2 + q3) + 3*q2_dot*q3_dotdot*sin(q1 + q2 + q3) + 3*q3_dot*q2_dotdot*sin(q1 + q2 + q3) + 3*q3_dot*q3_dotdot*sin(q1 + q2 + q3) + 3*q1_dot*q2_dot^2*cos(q1 + q2 + q3) + 3*q1_dot^2*q2_dot*cos(q1 + q2 + q3) + 3*q1_dot*q3_dot^2*cos(q1 + q2 + q3) + 3*q1_dot^2*q3_dot*cos(q1 + q2 + q3) + 3*q2_dot*q3_dot^2*cos(q1 + q2 + q3) + 3*q2_dot^2*q3_dot*cos(q1 + q2 + q3) + 3*q1_dot*q1_dotdot*sin(q1 + q2) + 3*q1_dot*q2_dotdot*sin(q1 + q2) + 3*q2_dot*q1_dotdot*sin(q1 + q2) + 3*q2_dot*q2_dotdot*sin(q1 + q2) + 6*q1_dot*q2_dot*q3_dot*cos(q1 + q2 + q3), q1_dot^3*cos(q1 + q2 + q3) + q2_dot^3*cos(q1 + q2 + q3) + q3_dot^3*cos(q1 + q2 + q3) - q1_tridot*cos(q1 + q2) - q2_tridot*cos(q1 + q2) + q1_dot^3*cos(q1 + q2) + q2_dot^3*cos(q1 + q2) - q1_tridot*cos(q1 + q2 + q3) - q2_tridot*cos(q1 + q2 + q3) - q3_tridot*cos(q1 + q2 + q3) + 3*q1_dot*q2_dot^2*cos(q1 + q2) + 3*q1_dot^2*q2_dot*cos(q1 + q2) + 3*q1_dot*q1_dotdot*sin(q1 + q2 + q3) + 3*q1_dot*q2_dotdot*sin(q1 + q2 + q3) + 3*q2_dot*q1_dotdot*sin(q1 + q2 + q3) + 3*q1_dot*q3_dotdot*sin(q1 + q2 + q3) + 3*q2_dot*q2_dotdot*sin(q1 + q2 + q3) + 3*q3_dot*q1_dotdot*sin(q1 + q2 + q3) + 3*q2_dot*q3_dotdot*sin(q1 + q2 + q3) + 3*q3_dot*q2_dotdot*sin(q1 + q2 + q3) + 3*q3_dot*q3_dotdot*sin(q1 + q2 + q3) + 3*q1_dot*q2_dot^2*cos(q1 + q2 + q3) + 3*q1_dot^2*q2_dot*cos(q1 + q2 + q3) + 3*q1_dot*q3_dot^2*cos(q1 + q2 + q3) + 3*q1_dot^2*q3_dot*cos(q1 + q2 + q3) + 3*q2_dot*q3_dot^2*cos(q1 + q2 + q3) + 3*q2_dot^2*q3_dot*cos(q1 + q2 + q3) + 3*q1_dot*q1_dotdot*sin(q1 + q2) + 3*q1_dot*q2_dotdot*sin(q1 + q2) + 3*q2_dot*q1_dotdot*sin(q1 + q2) + 3*q2_dot*q2_dotdot*sin(q1 + q2) + 6*q1_dot*q2_dot*q3_dot*cos(q1 + q2 + q3), q1_dot^3*cos(q1 + q2 + q3) + q2_dot^3*cos(q1 + q2 + q3) + q3_dot^3*cos(q1 + q2 + q3) - q1_tridot*cos(q1 + q2 + q3) - q2_tridot*cos(q1 + q2 + q3) - q3_tridot*cos(q1 + q2 + q3) + 3*q1_dot*q1_dotdot*sin(q1 + q2 + q3) + 3*q1_dot*q2_dotdot*sin(q1 + q2 + q3) + 3*q2_dot*q1_dotdot*sin(q1 + q2 + q3) + 3*q1_dot*q3_dotdot*sin(q1 + q2 + q3) + 3*q2_dot*q2_dotdot*sin(q1 + q2 + q3) + 3*q3_dot*q1_dotdot*sin(q1 + q2 + q3) + 3*q2_dot*q3_dotdot*sin(q1 + q2 + q3) + 3*q3_dot*q2_dotdot*sin(q1 + q2 + q3) + 3*q3_dot*q3_dotdot*sin(q1 + q2 + q3) + 3*q1_dot*q2_dot^2*cos(q1 + q2 + q3) + 3*q1_dot^2*q2_dot*cos(q1 + q2 + q3) + 3*q1_dot*q3_dot^2*cos(q1 + q2 + q3) + 3*q1_dot^2*q3_dot*cos(q1 + q2 + q3) + 3*q2_dot*q3_dot^2*cos(q1 + q2 + q3) + 3*q2_dot^2*q3_dot*cos(q1 + q2 + q3) + 6*q1_dot*q2_dot*q3_dot*cos(q1 + q2 + q3);
q1_dot^3*sin(q1) + q1_dot^3*sin(q1 + q2 + q3) + q2_dot^3*sin(q1 + q2 + q3) + q3_dot^3*sin(q1 + q2 + q3) - q1_tridot*sin(q1 + q2) - q2_tridot*sin(q1 + q2) - q1_tridot*sin(q1) + q1_dot^3*sin(q1 + q2) + q2_dot^3*sin(q1 + q2) - q1_tridot*sin(q1 + q2 + q3) - q2_tridot*sin(q1 + q2 + q3) - q3_tridot*sin(q1 + q2 + q3) - 3*q1_dot*q1_dotdot*cos(q1) + 3*q1_dot*q2_dot^2*sin(q1 + q2) + 3*q1_dot^2*q2_dot*sin(q1 + q2) - 3*q1_dot*q1_dotdot*cos(q1 + q2 + q3) - 3*q1_dot*q2_dotdot*cos(q1 + q2 + q3) - 3*q2_dot*q1_dotdot*cos(q1 + q2 + q3) - 3*q1_dot*q3_dotdot*cos(q1 + q2 + q3) - 3*q2_dot*q2_dotdot*cos(q1 + q2 + q3) - 3*q3_dot*q1_dotdot*cos(q1 + q2 + q3) - 3*q2_dot*q3_dotdot*cos(q1 + q2 + q3) - 3*q3_dot*q2_dotdot*cos(q1 + q2 + q3) - 3*q3_dot*q3_dotdot*cos(q1 + q2 + q3) + 3*q1_dot*q2_dot^2*sin(q1 + q2 + q3) + 3*q1_dot^2*q2_dot*sin(q1 + q2 + q3) + 3*q1_dot*q3_dot^2*sin(q1 + q2 + q3) + 3*q1_dot^2*q3_dot*sin(q1 + q2 + q3) + 3*q2_dot*q3_dot^2*sin(q1 + q2 + q3) + 3*q2_dot^2*q3_dot*sin(q1 + q2 + q3) - 3*q1_dot*q1_dotdot*cos(q1 + q2) - 3*q1_dot*q2_dotdot*cos(q1 + q2) - 3*q2_dot*q1_dotdot*cos(q1 + q2) - 3*q2_dot*q2_dotdot*cos(q1 + q2) + 6*q1_dot*q2_dot*q3_dot*sin(q1 + q2 + q3), q1_dot^3*sin(q1 + q2 + q3) + q2_dot^3*sin(q1 + q2 + q3) + q3_dot^3*sin(q1 + q2 + q3) - q1_tridot*sin(q1 + q2) - q2_tridot*sin(q1 + q2) + q1_dot^3*sin(q1 + q2) + q2_dot^3*sin(q1 + q2) - q1_tridot*sin(q1 + q2 + q3) - q2_tridot*sin(q1 + q2 + q3) - q3_tridot*sin(q1 + q2 + q3) + 3*q1_dot*q2_dot^2*sin(q1 + q2) + 3*q1_dot^2*q2_dot*sin(q1 + q2) - 3*q1_dot*q1_dotdot*cos(q1 + q2 + q3) - 3*q1_dot*q2_dotdot*cos(q1 + q2 + q3) - 3*q2_dot*q1_dotdot*cos(q1 + q2 + q3) - 3*q1_dot*q3_dotdot*cos(q1 + q2 + q3) - 3*q2_dot*q2_dotdot*cos(q1 + q2 + q3) - 3*q3_dot*q1_dotdot*cos(q1 + q2 + q3) - 3*q2_dot*q3_dotdot*cos(q1 + q2 + q3) - 3*q3_dot*q2_dotdot*cos(q1 + q2 + q3) - 3*q3_dot*q3_dotdot*cos(q1 + q2 + q3) + 3*q1_dot*q2_dot^2*sin(q1 + q2 + q3) + 3*q1_dot^2*q2_dot*sin(q1 + q2 + q3) + 3*q1_dot*q3_dot^2*sin(q1 + q2 + q3) + 3*q1_dot^2*q3_dot*sin(q1 + q2 + q3) + 3*q2_dot*q3_dot^2*sin(q1 + q2 + q3) + 3*q2_dot^2*q3_dot*sin(q1 + q2 + q3) - 3*q1_dot*q1_dotdot*cos(q1 + q2) - 3*q1_dot*q2_dotdot*cos(q1 + q2) - 3*q2_dot*q1_dotdot*cos(q1 + q2) - 3*q2_dot*q2_dotdot*cos(q1 + q2) + 6*q1_dot*q2_dot*q3_dot*sin(q1 + q2 + q3), q1_dot^3*sin(q1 + q2 + q3) + q2_dot^3*sin(q1 + q2 + q3) + q3_dot^3*sin(q1 + q2 + q3) - q1_tridot*sin(q1 + q2 + q3) - q2_tridot*sin(q1 + q2 + q3) - q3_tridot*sin(q1 + q2 + q3) - 3*q1_dot*q1_dotdot*cos(q1 + q2 + q3) - 3*q1_dot*q2_dotdot*cos(q1 + q2 + q3) - 3*q2_dot*q1_dotdot*cos(q1 + q2 + q3) - 3*q1_dot*q3_dotdot*cos(q1 + q2 + q3) - 3*q2_dot*q2_dotdot*cos(q1 + q2 + q3) - 3*q3_dot*q1_dotdot*cos(q1 + q2 + q3) - 3*q2_dot*q3_dotdot*cos(q1 + q2 + q3) - 3*q3_dot*q2_dotdot*cos(q1 + q2 + q3) - 3*q3_dot*q3_dotdot*cos(q1 + q2 + q3) + 3*q1_dot*q2_dot^2*sin(q1 + q2 + q3) + 3*q1_dot^2*q2_dot*sin(q1 + q2 + q3) + 3*q1_dot*q3_dot^2*sin(q1 + q2 + q3) + 3*q1_dot^2*q3_dot*sin(q1 + q2 + q3) + 3*q2_dot*q3_dot^2*sin(q1 + q2 + q3) + 3*q2_dot^2*q3_dot*sin(q1 + q2 + q3) + 6*q1_dot*q2_dot*q3_dot*sin(q1 + q2 + q3)];





p_in=[1.41;-0.41];
p_fin=[1.41;0.41];

h=norm(p_fin-p_in);
T=2.58;

s=h*(-20*(t/T)^7+70*(t/T)^6-84*(t/T)^5+35*(t/T)^4);

s_1=140*h/T*(-(t/T)^6+3*(t/T)^5-3*(t/T)^4+(t/T)^3);

s_2=420*h/T^2*(-2*(t/T)^5+5*(t/T)^4-4*(t/T)^3+(t/T)^2);

s_3=840*h/T^3*(-5*(t/T)^4+10*(t/T)^3-6*(t/T)^2+(t/T));

s_4=840*h/T^4*(-20*(t/T)^3+30*(t/T)^2-12*(t/T)+1);


r=p_in+s/h*(p_fin-p_in);

r_1=s_1/h*(p_fin-p_in);

r_2=s_2/h*(p_fin-p_in);
 
r_3=s_3/h*(p_fin-p_in);

r_4=s_4/h*(p_fin-p_in);

p_3=J*q_triplodot+2*Jdot*qdotdot+Jdotdot*qdot;
p_2=Jdot*qdot+J*qdotdot;
p_1=J*qdot;

% caso con (s+10)^2*(s+5)^2
K_0=2500*eye(2);
K_1=1500*eye(2);
K_2=325*eye(2);
K_3=30*eye(2);



X=r_4+K_3*(r_3-p_3)+K_2*(r_2-p_2)+K_1*(r_1-p_1)+K_0*(r-p);

y = X-3*Jdot*[q1_tridot;q2_tridot;q3_tridot]-2*Jdotdot*[q1_dotdot;q2_dotdot;q3_dotdot]-Jtriplodot*[q1_dot;q2_dot;q3_dot];

== matlab function Progetto_robotics_linear/ c(q,qdot) ==
  data: q input; y output; qdot input
function y = fcn(q,qdot)


q1=q(1);
q2=q(2);
q3=q(3);

q1_dot=qdot(1);
q2_dot=qdot(2);
q3_dot=qdot(3);




c=[- q1_dot*(q3_dot*(5*sin(q2 + q3) + 5*sin(q3)) + q2_dot*(5*sin(q2 + q3) + 16*sin(q2))) - q3_dot*(q1_dot*(5*sin(q2 + q3) + 5*sin(q3)) + q2_dot*(5*sin(q2 + q3) + 5*sin(q3)) + q3_dot*(5*sin(q2 + q3) + 5*sin(q3))) - q2_dot*(q3_dot*(5*sin(q2 + q3) + 5*sin(q3)) + q2_dot*(5*sin(q2 + q3) + 11*sin(q2)) + q1_dot*(5*sin(q2 + q3) + 16*sin(q2)));
                                                                                                                                                                                q1_dot*(q1_dot*(5*sin(q2 + q3) + 16*sin(q2)) - 5*q3_dot*sin(q3)) - q3_dot*(5*q1_dot*sin(q3) + 5*q2_dot*sin(q3) + 10*q3_dot*sin(q3)) - 5*q2_dot*q3_dot*sin(q3);
                                                                                                                                                                                                                               q1_dot*(q1_dot*(5*sin(q2 + q3) + 5*sin(q3)) + 5*q2_dot*sin(q3)) + q2_dot*(5*q1_dot*sin(q3) + 5*q2_dot*sin(q3))];
                                                                                                                                                                                                                                                                                                                                                         
                                                                                                                                                                                                                                                                                                                                                            
                                                                                                                                                                                                                                                                                                                                                            
y = c;

== matlab function Progetto_robotics_linear/  M_inversa ==
  data: q input; qdotdot output; ingresso input
function qdotdot = M_inversa(q,ingresso)


q1=q(1);
q2=q(2);
q3=q(3);
M=[10*cos(q2 + q3) + 32*cos(q2) + 10*cos(q3) + 5049/100, 5*cos(q2 + q3) + 11*cos(q2) + 10*cos(q3) + 504/25, 5*cos(q2 + q3) + 5*cos(q3) + 583/100;
   5*cos(q2 + q3) + 11*cos(q2) + 10*cos(q3) + 504/25,                              10*cos(q3) + 1133/50,                 10*cos(q3) + 583/100;
                5*cos(q2 + q3) + 5*cos(q3) + 583/100,                              10*cos(q3) + 583/100,                              583/100];




qdotdot = inv(M)*ingresso;

== matlab function Progetto_robotics_linear/torque ==
  data: q input; tau output; q_quattrodot input; alpha input; gain input
function tau = fcn(q,q_quattrodot,alpha,gain)
B=100*[1,0,0;
    0,1,0;
    0,0,1];
K=gain*eye(3);

q1=q(1);
q2=q(2);
q3=q(3);

M=[10*cos(q2 + q3) + 32*cos(q2) + 10*cos(q3) + 5049/100, 5*cos(q2 + q3) + 11*cos(q2) + 10*cos(q3) + 504/25, 5*cos(q2 + q3) + 5*cos(q3) + 583/100;
   5*cos(q2 + q3) + 11*cos(q2) + 10*cos(q3) + 504/25,                              10*cos(q3) + 1133/50,                 10*cos(q3) + 583/100;
                5*cos(q2 + q3) + 5*cos(q3) + 583/100,                              10*cos(q3) + 583/100,                              583/100];




tau = B*inv(K)*(M*q_quattrodot+alpha);
